simulink model "aufgabe1_mod"  (R2018b)
settings: Solver=VariableStepAuto  StartTime=0.0  StopTime=10  RelTol=1e-3
values from neighbouring files (symbols this model uses):
  Kd = 0.125*Tkrit*Kp    (= 1.026)    [Aufgabe1.m]
  Ki = 2/Tkrit*Kp    (= 4.54736842105)    [Aufgabe1.m]
  Kp = 0.6*Kkrit    (= 4.32)    [Aufgabe1.m]
  p1 = -1    [Aufgabe1.m]
  p2 = -0.5    [Aufgabe1.m]
  T1 = 0.001    [Aufgabe1.m]
settings Model: Creator=Peter  LastModifiedBy=Peter

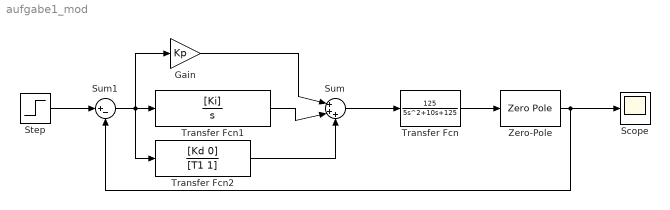
== system aufgabe1_mod ==
  Gain : Gain  Gain=Kp
  Scope : Scope
  Step : Step  SampleTime=0
  Sum : Sum  Inputs=|+++
  Sum1 : Sum  Inputs=|+-
  Transfer Fcn : TransferFcn  Numerator=[125]  Denominator=[5 10 125]
  Transfer Fcn1 : TransferFcn  Numerator=[Ki]  Denominator=[1 0]
  Transfer Fcn2 : TransferFcn  Numerator=[Kd 0]  Denominator=[T1 1]
  Zero-Pole : ZeroPole  Zeros=[]  Poles=[p1 p2]
  wires:
  Transfer Fcn/1 -> Zero-Pole/1
  Gain/1 -> Sum/1
  Transfer Fcn1/1 -> Sum/2
  Transfer Fcn2/1 -> Sum/3
  Step/1 -> Sum1/1
  Sum1/1 -> Transfer Fcn2/1, Gain/1, Transfer Fcn1/1
  Sum/1 -> Transfer Fcn/1
  Zero-Pole/1 -> Sum1/2, Scope/1
